simulink model "Full_System"  (R2025b)
settings: Solver=VariableStepAuto  StartTime=0.0  StopTime=10.0  RelTol=1e-3
settings Model: Creator=koryh  LastModifiedBy=koryh

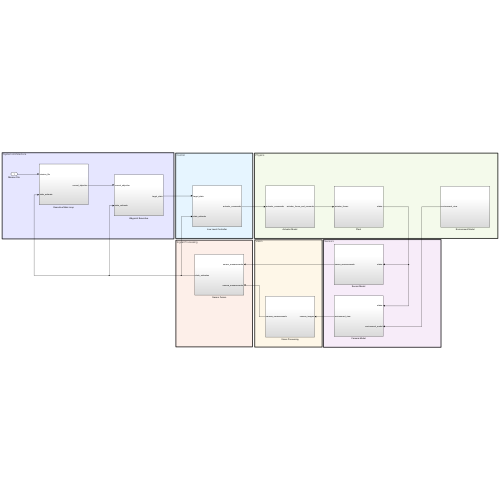
[thumbnail: Simulink's stored preview of the top-level diagram]
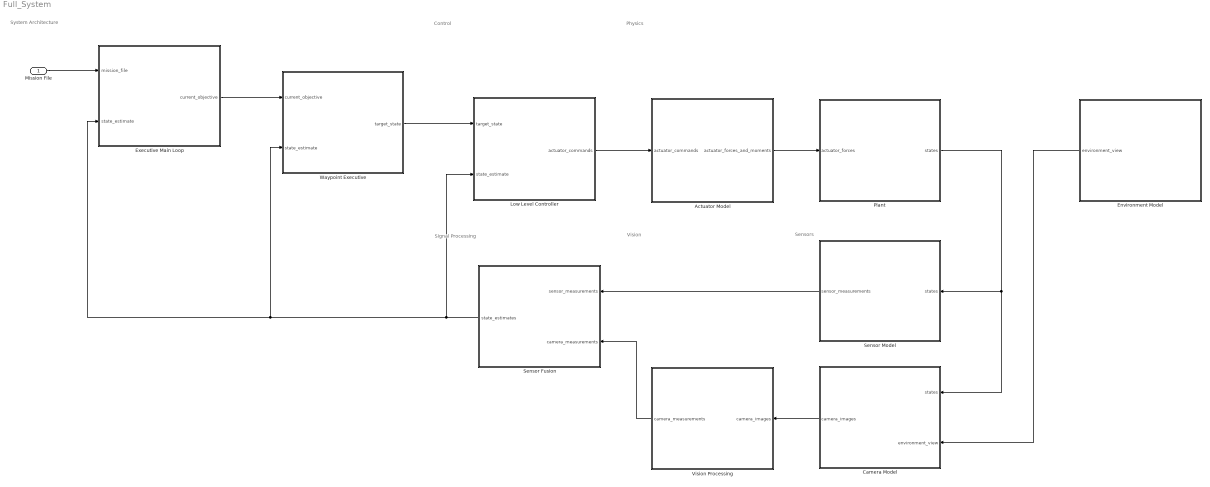
== system Full_System ==
  note: Signal Processing
  note: Vision
  note: Sensors
  note: Physics
  note: Control
  note: System Architecture
  Mission File : Inport
  Actuator Model : Subsystem
  Camera Model : Subsystem
  Environment Model : Subsystem
  Executive Main Loop : Subsystem
  Low Level Controller : Subsystem
  Plant : Subsystem
  Sensor Fusion : Subsystem
  Sensor Model : Subsystem
  Vision Processing : Subsystem
  Waypoint Executive : Subsystem
  wires:
  Mission File/1 -> Executive Main Loop/1(mission_file)
  Executive Main Loop/1(current_objective) -> Waypoint Executive/1(current_objective)
  Waypoint Executive/1(target_state) -> Low Level Controller/1(target_state)
  Low Level Controller/1(actuator_commands) -> Actuator Model/1(actuator_commands)
  Actuator Model/1(actuator_forces_and_moments) -> Plant/1(actuator_forces)
  Plant/1(states) -> Sensor Model/1(states), Camera Model/1(states)
  Environment Model/1(environment_view) -> Camera Model/2(environment_view)
  Camera Model/1(camera_images) -> Vision Processing/1(camera_images)
  Sensor Model/1(sensor_measurements) -> Sensor Fusion/1(sensor_measurements)
  Vision Processing/1(camera_measurements) -> Sensor Fusion/2(camera_measurements)
  Sensor Fusion/1(state_estimates) -> Waypoint Executive/2(state_estimate), Executive Main Loop/2(state_estimate), Low Level Controller/2(state_estimate)

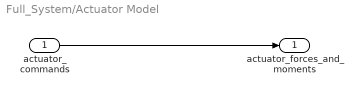
== system Full_System/Actuator Model ==
  actuator_commands : Inport
  actuator_forces_and_moments : Outport
  wires:
  actuator_commands/1 -> actuator_forces_and_moments/1

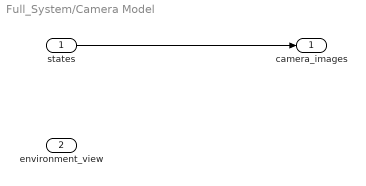
== system Full_System/Camera Model ==
  states : Inport
  environment_view : Inport  Port=2
  camera_images : Outport
  wires:
  states/1 -> camera_images/1

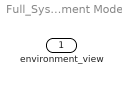
== system Full_System/Environment Model ==
  environment_view : Outport

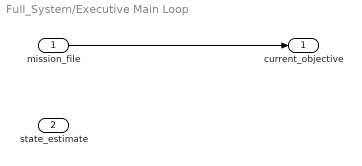
== system Full_System/Executive Main Loop ==
  mission_file : Inport
  state_estimate : Inport  Port=2
  current_objective : Outport
  wires:
  mission_file/1 -> current_objective/1

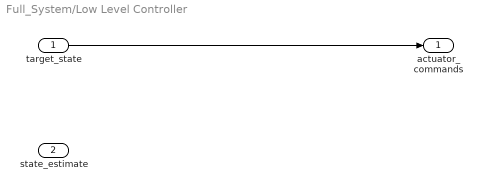
== system Full_System/Low Level Controller ==
  target_state : Inport
  state_estimate : Inport  Port=2
  actuator_commands : Outport
  wires:
  target_state/1 -> actuator_commands/1

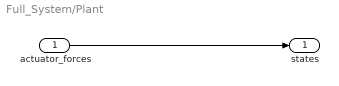
== system Full_System/Plant ==
  actuator_forces : Inport
  states : Outport
  wires:
  actuator_forces/1 -> states/1

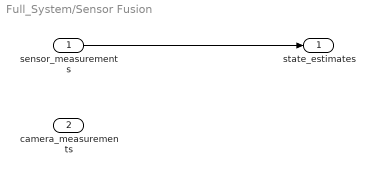
== system Full_System/Sensor Fusion ==
  sensor_measurements : Inport
  camera_measurements : Inport  Port=2
  state_estimates : Outport
  wires:
  sensor_measurements/1 -> state_estimates/1

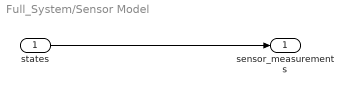
== system Full_System/Sensor Model ==
  states : Inport
  sensor_measurements : Outport
  wires:
  states/1 -> sensor_measurements/1

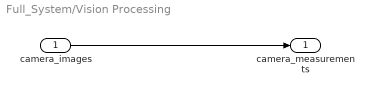
== system Full_System/Vision Processing ==
  camera_images : Inport
  camera_measurements : Outport
  wires:
  camera_images/1 -> camera_measurements/1

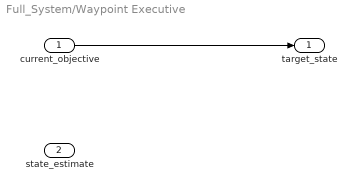
== system Full_System/Waypoint Executive ==
  current_objective : Inport
  state_estimate : Inport  Port=2
  target_state : Outport
  wires:
  current_objective/1 -> target_state/1
